simulink model "Full_car_model_build_Rajesh_Ramani_textbook"  (R2024b)
settings: Solver=VariableStepAuto  StartTime=0.0  StopTime=10  RelTol=1e-3
model workspace: external: MATLAB File C:\Users\USER\Documents\MATLAB\NR\TV_lisb_helper_file.m (data not in the file)
values from neighbouring files (symbols this model uses):
  g = 9.8    [TV_lisb_helper_file.m]
  hCG = 0.6    [TV_lisb_helper_file.m]
  Izz = 3000    [TV_lisb_helper_file.m]
  lf = 1.5    [TV_lisb_helper_file.m]
  lr = 1.5    [TV_lisb_helper_file.m]
  M = 300    [TV_lisb_helper_file.m]
  tr = 1    [TV_lisb_helper_file.m]
libraries: autolibshared x4
(part 1 of 4)
settings Model: Creator=USER  LastModifiedBy=USER

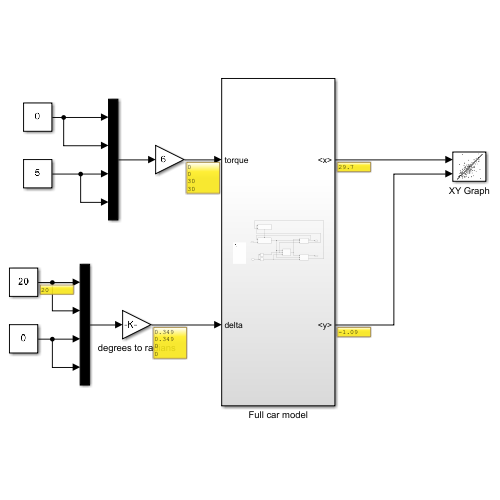
[thumbnail: Simulink's stored preview of the top-level diagram]
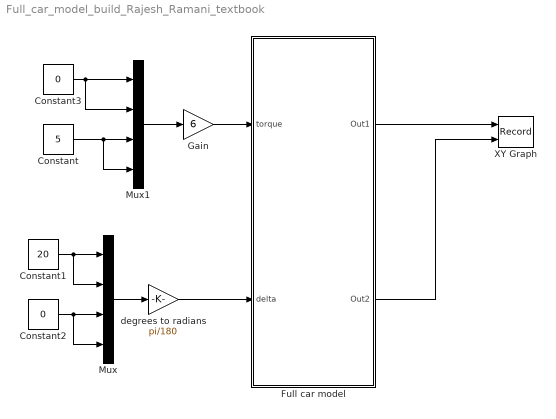
== system Full_car_model_build_Rajesh_Ramani_textbook ==
  Constant : Constant  Value=5
  Constant1 : Constant  Value=20
  Constant2 : Constant  Value=0
  Constant3 : Constant  Value=0
  Full car model : Subsystem
  Gain : Gain  Gain=6
  Mux : Mux
  Mux1 : Mux
  XY Graph : Record  FileSettingsInternal="{\"entries\":[{\"content\":{\"excelSettings\":{\"content\":{},\"type\":\"Streamout.ExcelSettings\"}},\"type\":\"Streamout.FileSettingStorage\",\"uuid\":\"\"}],\"packageUris\":[\"http:\\/\\/schema.mathworks.com\\/mf0\\/streamout_blocks\\/R2020a\"],\"version\":\"1.0\"}"  Layout=[1 1]  SignalsInternal="{\"entries\":[{\"content\":{\"signals\":[{\"content\":{\"blockPath\":[],\"dimensions\":[1],\"domain\":\"\",\"lineColor\":\"#ff6929\",\"lineWidth\":2,\"plots\":[ 1 ],\"port\":1,\"sid\":[\"\"],\"signalID\":1,\"signalName\":\"Full car model:1\"},\"type\":\"RecordBlkView.Signal\",\"uuid\":\"\"},{\"content\":{\"blockPath\":[],\"dimensions\":[1],\"domain\":\"\",\"lineColor\":\"#ff13a6\",\"lineWidth\":2,\"plots\":[ 1 ],\"port\":2,\"sid\":[\"\"],\"signalID\":2,\"signalName\":\"Full car model:2\"},\"type\":\"RecordBlkView.Signal\",\"uuid\":\"\"}]},\"type\":\"RecordBlkView.InputSignals\",\"uuid\":\"\"}],\"packageUris\":[\"http:\\/\\/schema.mathworks.com\\/mf0\\/streamout_blocks\\/R2020a\"],\"version\":\"1.0\"}"  VisualizationBindings="{\"xyplotplugin\":{\"info\":[{\"series\":[{\"bindingParametersList\":[{\"parameter\":\"X-Axis\",\"signalID\":1,\"signalName\":\"Full car model:1\"},{\"parameter\":\"Y-Axis\",\"signalID\":2,\"signalName\":\"Full car model:2\"},{\"parameter\":\"X-Axis\",\"signalID\":1,\"signalName\":\"Full car model:1\"},{\"parameter\":\"Y-Axis\",\"signalID\":2,\"signalName\":\"Full car model:2\"},{\"parameter\":\"X-Axis\",\"signalID\":1,\"signalName\":\"Full car model:1\"},{\"parameter\":\"Y-Axis\",\"signalID\":2,\"signalName\":\"Full car model:2\"},{\"parameter\":\"X-Axis\",\"signalID\":1,\"signalName\":\"Full car model:1\"},{\"parameter\":\"Y-Axis\",\"signalID\":2,\"signalName\":\"Full car model:2\"}],\"seriesID\":0}],\"subplotID\":1}]}}"  CompatibilityTag=XY
  degrees to radians : Gain  Gain=pi/180
  wires:
  Mux1/1 -> Gain/1
  Gain/1 -> Full car model/1(torque)
  degrees to radians/1 -> Full car model/2(delta)
  Full car model/1(Out1) -> XY Graph/1
  Full car model/2(Out2) -> XY Graph/2
  Mux/1 -> degrees to radians/1
  Constant1/1 -> Mux/2, Mux/1
  Constant2/1 -> Mux/4, Mux/3
  Constant/1 -> Mux1/4, Mux1/3
  Constant3/1 -> Mux1/2, Mux1/1

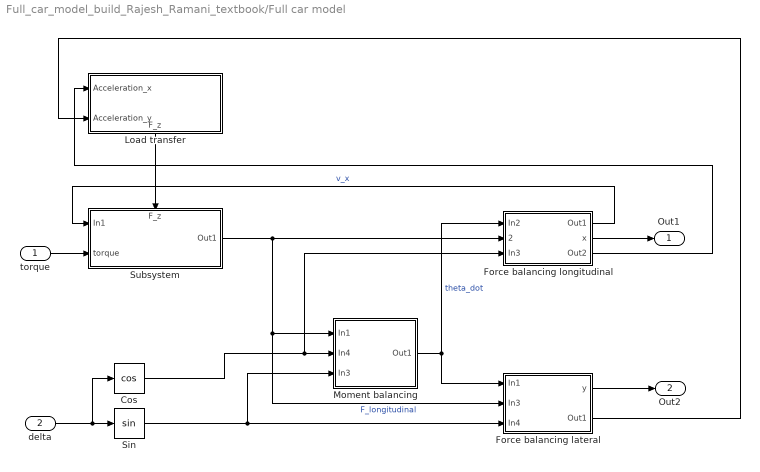
== system Full_car_model_build_Rajesh_Ramani_textbook/Full car model ==
  torque : Inport
  delta : Inport  Port=2
  Cos : Trigonometry  Operator=cos
  Force balancing lateral : Subsystem
  Force balancing longitudinal : Subsystem
  Load transfer : Subsystem
      settings: PortSchema="{\"entries\":[{\"content\":{\"sides\":[{\"content\":{\"connectorIds\":[\"In1\",\"In2\"]},\"type\":\"ConnectorPlacement.EquallySpacedRectSide\",\"uuid\":\"7a92a029-f41c-4e83-8aa5-ec6ce698d097\"},{\"content\":{\"side\":\"RIGHT\"},\"type\":\"ConnectorPlacement.EquallySpacedRectSide\",\"uuid\":\"18898237-2ea1-4fb3-bf3b-8bf473bf92ef\"},{\"content\":{\"side\":\"TOP\"},\"type\":\"ConnectorPlacement.EquallySpacedRectSide\",\"uuid\":\"0d9cde28-1c95-4b87-bc51-b880830b2cd8\"},{\"content\":{\"connectorIds\":[\"Out1\"],\"side\":\"BOTTOM\"},\"type\":\"ConnectorPlacement.EquallySpacedRectSide\",\"uuid\":\"5775db67-e45f-4ef5-9bbc-0ac2bf107565\"}]},\"type\":\"ConnectorPlacement.EquallySpacedConnector\",\"uuid\":\"13699207-135e-4293-942d-a225480078cb\"}],\"packageUris\":[\"http://schema.mathworks.com/mf0/Connector/R2020b\"],\"version\":\"1.0\"}"
  Moment balancing : Subsystem
  Sin : Trigonometry
  Subsystem : Subsystem
      settings: PortSchema="{\"entries\":[{\"content\":{\"sides\":[{\"content\":{\"connectorIds\":[\"In1\",\"In2\"]},\"type\":\"ConnectorPlacement.EquallySpacedRectSide\",\"uuid\":\"7a92a029-f41c-4e83-8aa5-ec6ce698d097\"},{\"content\":{\"connectorIds\":[\"Out1\"],\"side\":\"RIGHT\"},\"type\":\"ConnectorPlacement.EquallySpacedRectSide\",\"uuid\":\"18898237-2ea1-4fb3-bf3b-8bf473bf92ef\"},{\"content\":{\"connectorIds\":[\"In3\"],\"side\":\"TOP\"},\"type\":\"ConnectorPlacement.EquallySpacedRectSide\",\"uuid\":\"0d9cde28-1c95-4b87-bc51-b880830b2cd8\"}]},\"type\":\"ConnectorPlacement.EquallySpacedConnector\",\"uuid\":\"13699207-135e-4293-942d-a225480078cb\"}],\"packageUris\":[\"http://schema.mathworks.com/mf0/Connector/R2020b\"],\"version\":\"1.0\"}"
  Out1 : Outport
  Out2 : Outport  Port=2
  wires:
  delta/1 -> Sin/1, Cos/1
  Moment balancing/1(Out1) -> Force balancing longitudinal/1(In2), Force balancing lateral/1(In1)  "theta_dot"
  Cos/1 -> Force balancing longitudinal/3(In3), Moment balancing/2(In4)
  Subsystem/1(Out1) -> Moment balancing/1(In1), Force balancing lateral/2(In3), Force balancing longitudinal/2(2)  "F_longitudinal"
  Sin/1 -> Moment balancing/3(In3), Force balancing lateral/3(In4)
  Force balancing longitudinal/2(x) -> Out1/1
  Force balancing lateral/1(y) -> Out2/1
  torque/1 -> Subsystem/2(torque)
  Force balancing longitudinal/1(Out1) -> Subsystem/1(In1)  "v_x"
  Force balancing longitudinal/3(Out2) -> Load transfer/1(Acceleration_x)
  Force balancing lateral/2(Out1) -> Load transfer/2(Acceleration_y)
  Load transfer/1(F_z) -> Subsystem/3(F_z)

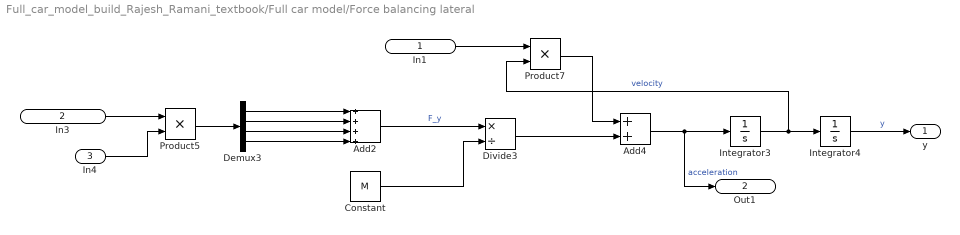
== system Full_car_model_build_Rajesh_Ramani_textbook/Full car model/Force balancing lateral ==
  In1 : Inport
  In3 : Inport  Port=2
  In4 : Inport  Port=3
  Add2 : Sum  Inputs=++++
  Add4 : Sum
  Constant : Constant  Value=M
  Demux3 : Demux
  Divide3 : Product  Inputs=*/
  Integrator3 : Integrator
  Integrator4 : Integrator
  Product5 : Product
  Product7 : Product
  y : Outport
  Out1 : Outport  Port=2
  wires:
  Integrator3/1 -> Product7/2, Integrator4/1  "velocity"
  Demux3/1 -> Add2/1
  Add2/1 -> Divide3/1  "F_y"
  Product7/1 -> Add4/1
  Divide3/1 -> Add4/2
  Demux3/2 -> Add2/2
  Add4/1 -> Out1/1, Integrator3/1  "acceleration"
  Demux3/4 -> Add2/4
  Demux3/3 -> Add2/3
  In4/1 -> Product5/2
  Product5/1 -> Demux3/1
  In1/1 -> Product7/1
  In3/1 -> Product5/1
  Integrator4/1 -> y/1  "y"
  Constant/1 -> Divide3/2

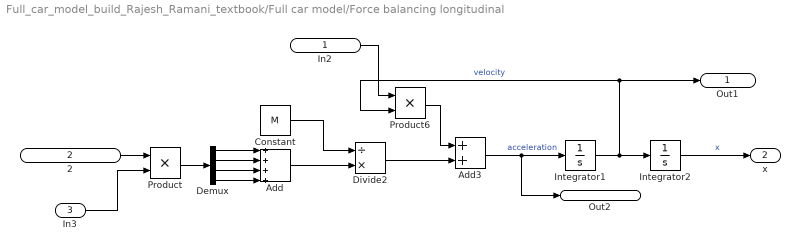
== system Full_car_model_build_Rajesh_Ramani_textbook/Full car model/Force balancing longitudinal ==
  In2 : Inport
  2 : Inport  Port=2
  In3 : Inport  Port=3
  Add : Sum  Inputs=++++
  Add3 : Sum
  Constant : Constant  Value=M
  Demux : Demux
  Divide2 : Product  Inputs=/*
  Integrator1 : Integrator
  Integrator2 : Integrator
  Product : Product
  Product6 : Product
  Out1 : Outport
  x : Outport  Port=2
  Out2 : Outport  Port=3
  wires:
  Product6/1 -> Add3/1
  Divide2/1 -> Add3/2
  Integrator1/1 -> Integrator2/1, Product6/2, Out1/1  "velocity"
  Add3/1 -> Out2/1, Integrator1/1  "acceleration"
  In2/1 -> Product6/1
  Constant/1 -> Divide2/1
  Integrator2/1 -> x/1  "x"
  Demux/1 -> Add/1
  Demux/2 -> Add/2
  Demux/3 -> Add/3
  Demux/4 -> Add/4
  Add/1 -> Divide2/2
  2/1 -> Product/1
  In3/1 -> Product/2
  Product/1 -> Demux/1

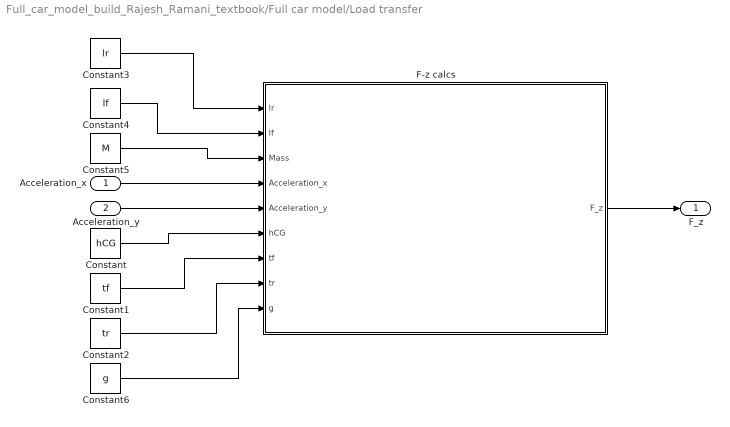
== system Full_car_model_build_Rajesh_Ramani_textbook/Full car model/Load transfer ==
  Acceleration_x : Inport
  Acceleration_y : Inport  Port=2
  Constant : Constant  Value=hCG
  Constant1 : Constant  Value=tf
  Constant2 : Constant  Value=tr
  Constant3 : Constant  Value=lr
  Constant4 : Constant  Value=lf
  Constant5 : Constant  Value=M
  Constant6 : Constant  Value=g
  F-z calcs : Subsystem
  F_z : Outport
  wires:
  F-z calcs/1(F_z) -> F_z/1
  Acceleration_x/1 -> F-z calcs/4(Acceleration_x)
  Acceleration_y/1 -> F-z calcs/5(Acceleration_y)
  Constant3/1 -> F-z calcs/1(lr)
  Constant4/1 -> F-z calcs/2(lf)
  Constant5/1 -> F-z calcs/3(Mass)
  Constant/1 -> F-z calcs/6(hCG)
  Constant1/1 -> F-z calcs/7(tf)
  Constant2/1 -> F-z calcs/8(tr)
  Constant6/1 -> F-z calcs/9(g)

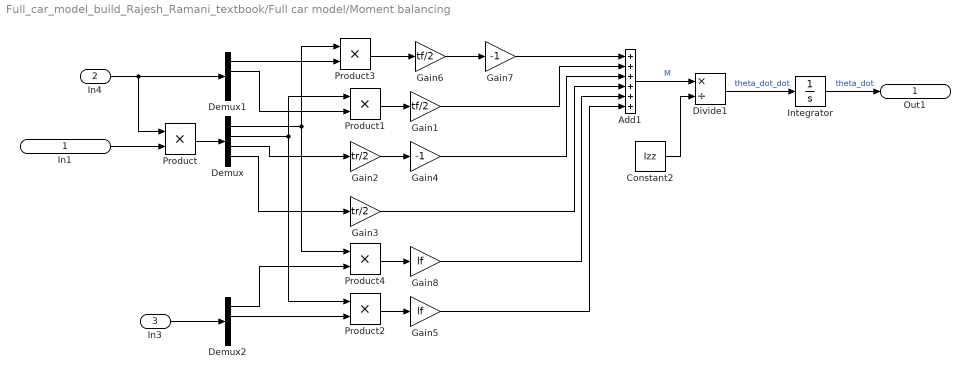
== system Full_car_model_build_Rajesh_Ramani_textbook/Full car model/Moment balancing ==
  In1 : Inport
  In4 : Inport  Port=2
  In3 : Inport  Port=3
  Add1 : Sum  Inputs=++++++
  Constant2 : Constant  Value=Izz
  Demux : Demux
  Demux1 : Demux
  Demux2 : Demux
  Divide1 : Product  Inputs=*/
  Gain1 : Gain  Gain=tf/2
  Gain2 : Gain  Gain=tr/2
  Gain3 : Gain  Gain=tr/2
  Gain4 : Gain  Gain=-1
  Gain5 : Gain  Gain=lf
  Gain6 : Gain  Gain=tf/2
  Gain7 : Gain  Gain=-1
  Gain8 : Gain  Gain=lf
  Integrator : Integrator
  Product{,1..4} (5 alike) : Product
  Out1 : Outport
  wires:
  Gain1/1 -> Add1/2
  Demux/3 -> Gain2/1
  Constant2/1 -> Divide1/2
  Demux/1 -> Product3/1, Product4/1
  Divide1/1 -> Integrator/1  "theta_dot_dot"
  Gain4/1 -> Add1/3
  Gain6/1 -> Gain7/1
  Demux/4 -> Gain3/1
  Add1/1 -> Divide1/1  "M"
  Product3/1 -> Gain6/1
  Gain7/1 -> Add1/1
  Demux2/1 -> Product4/2
  Product4/1 -> Gain8/1
  Demux/2 -> Product1/1, Product2/1
  Gain5/1 -> Add1/6
  Demux1/1 -> Product3/2
  Demux2/2 -> Product2/2
  Gain2/1 -> Gain4/1
  Product1/1 -> Gain1/1
  Demux1/2 -> Product1/2
  Gain8/1 -> Add1/5
  Gain3/1 -> Add1/4
  Product2/1 -> Gain5/1
  In4/1 -> Product/1, Demux1/1
  In3/1 -> Demux2/1
  Integrator/1 -> Out1/1  "theta_dot"
  Product/1 -> Demux/1
  In1/1 -> Product/2
